simulink model "Observador"  (R2019a)
settings: Solver=VariableStepAuto  StartTime=0.0  StopTime=5  RelTol=1e-3
values from neighbouring files (symbols this model uses):
  A = [0 1 0;42.5 0 20;0 0 -4]    [Berard_Modelo_ControlEE.m]
  B = [0 0 1]'    [Berard_Modelo_ControlEE.m]
  C = k*C    [Berard_LoopShaping.m]    (also in Berard_Modelo_ControlEE.m = [1 0 0])
  k_g = k_a(1:3)    [Berard_Modelo_ControlEE.m]
  k_i = -k_a(end)    [Berard_Modelo_ControlEE.m]
  L = R*C*H*M    [Berard_LoopShaping.m]    (also in Berard_Modelo_ControlEE.m = acker(A',C',[-70 -70 -70])')
settings Model: Creator=agusd  LastModifiedBy=ARLUBER1
settings DataIOCC: ReturnWorkspaceOutputs=off
settings DebuggingCC: ArithmeticOperatorsInVariantConditions=warning
settings SFSimCC: SimUseLocalCustomCode=off
settings RTWCC: RTWUseLocalCustomCode=off
settings CodeAppCC: StateflowObjectComments=on

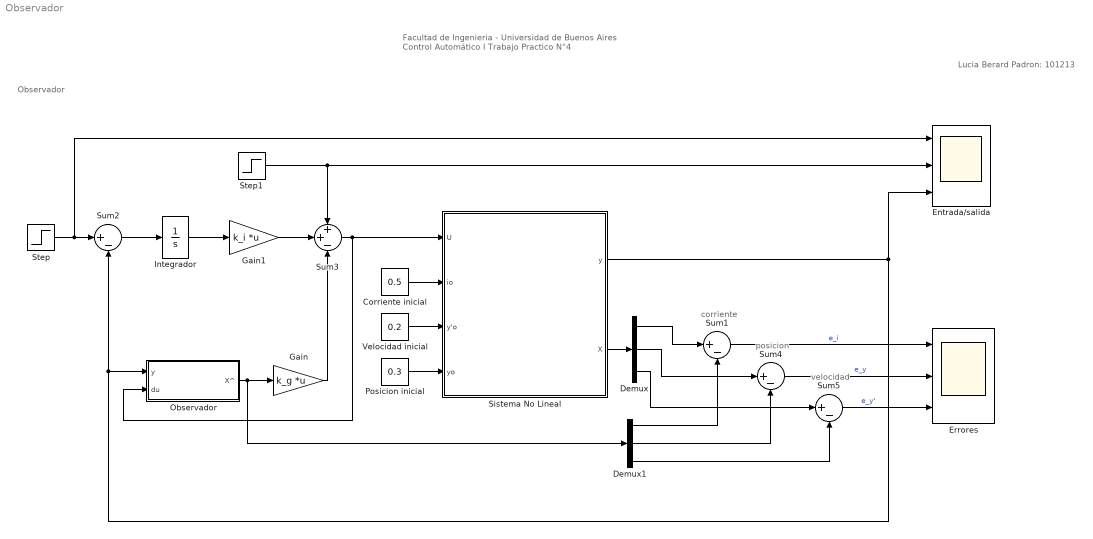
== system Observador ==
  note: velocidad
  note: posicion
  note: corriente
  note: Lucia Berard
      | Padron: 101213
  note: Observador
  note: Facultad de Ingenieria - Universidad de Buenos Aires
      | Control Automático I
      | Trabajo Practico N°4
  Corriente inicial : Constant  Value=0.5
  Demux : Demux  Outputs=3
  Demux1 : Demux  Outputs=3
  Entrada/salida : Scope  NumInputPorts=3
  Errores : Scope  NumInputPorts=3
  Gain : Gain  Gain=k_g  Multiplication=Matrix(K*u)
  Gain1 : Gain  Gain=k_i  Multiplication=Matrix(K*u)
  Integrador : Integrator
  Observador : Subsystem
  Posicion inicial : Constant  Value=0.3
  Sistema No Lineal : Subsystem
  Step : Step  After=0.5  SampleTime=0
  Step1 : Step  Time=3  After=0.55  SampleTime=0
  Sum{1..2,4..5} (4 alike) : Sum  Inputs=|+-
  Sum3 : Sum  Inputs=++-
  Velocidad inicial : Constant  Value=0.2
  wires:
  Corriente inicial/1 -> Sistema No Lineal/2(io)
  Velocidad inicial/1 -> Sistema No Lineal/3(y'o)
  Posicion inicial/1 -> Sistema No Lineal/4(yo)
  Step/1 -> Entrada/salida/1, Sum2/1
  Sum2/1 -> Integrador/1
  Integrador/1 -> Gain1/1
  Sum3/1 -> Observador/2(du), Sistema No Lineal/1(U)
  Sistema No Lineal/1("y ") -> Observador/1(y), Sum2/2, Entrada/salida/3
  Step1/1 -> Sum3/1, Entrada/salida/2
  Gain1/1 -> Sum3/2
  Observador/1(X^) -> Demux1/1, Gain/1
  Gain/1 -> Sum3/3
  Sum1/1 -> Errores/1  "e_i"
  Sum4/1 -> Errores/2  "e_y"
  Sum5/1 -> Errores/3  "e_y'"
  Sistema No Lineal/2(X) -> Demux/1
  Demux/1 -> Sum1/1
  Demux/2 -> Sum4/1
  Demux/3 -> Sum5/1
  Demux1/1 -> Sum1/2
  Demux1/2 -> Sum4/2
  Demux1/3 -> Sum5/2

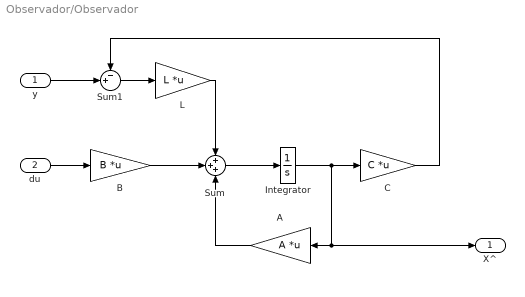
== system Observador/Observador ==
  y : Inport
  du : Inport  Port=2
  A : Gain  Gain=A  Multiplication=Matrix(K*u)
  B : Gain  Gain=B  Multiplication=Matrix(K*u)
  C : Gain  Gain=C  Multiplication=Matrix(K*u)
  Integrator : Integrator
  L : Gain  Gain=L  Multiplication=Matrix(K*u)
  Sum : Sum  Inputs=+++
  Sum1 : Sum  Inputs=-+|
  X^ : Outport
  wires:
  du/1 -> B/1
  Integrator/1 -> A/1, X^/1, C/1
  y/1 -> Sum1/2
  Sum1/1 -> L/1
  B/1 -> Sum/2
  A/1 -> Sum/3
  Sum/1 -> Integrator/1
  L/1 -> Sum/1
  C/1 -> Sum1/1

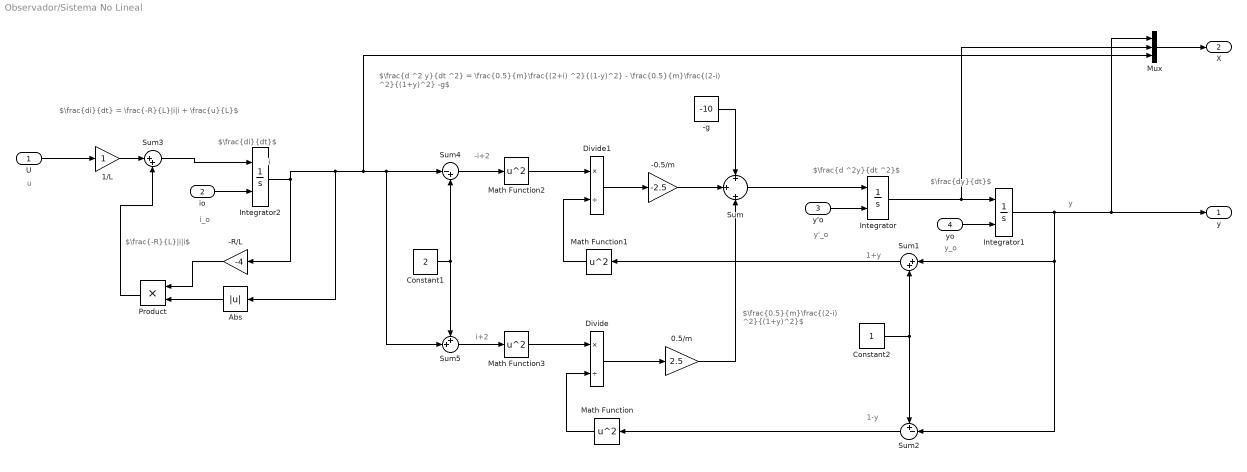
== system Observador/Sistema No Lineal ==
  note: y_o
  note: 1+y
  note: $\frac{di}{dt}$
  note: u
  note: i+2
  note: $\frac{d ^2 y}{dt ^2} = \frac{0.5}{m}\frac{(2+i) ^2}{(1-y)^2} - \frac{0.5}{m}\frac{(2-i) ^2}{(1+y)^2} -g$
  note: y
  note: 1-y
  note: i_o
  note: $\frac{dy}{dt}$
  note: y'_o
  note: $\frac{di}{dt} = \frac{-R}{L}|i|i + \frac{u}{L}$
  note: -i+2
  note: $\frac{-R}{L}|i|i$
  note: i
  note: $\frac{0.5}{m}\frac{(2-i) ^2}{(1+y)^2}$
  note: $\frac{d ^2y}{dt ^2}$
  U : Inport  OutDataTypeStr=double
  io : Inport  Port=2  OutDataTypeStr=double
  y'o : Inport  Port=3
  yo : Inport  Port=4
  -0.5/m : Gain  Gain=-2.5
  -R/L : Gain  Gain=-4
  -g : Constant  Value=-10
  0.5/m : Gain  Gain=2.5
  1/L : Gain
  Abs : Abs
  Constant1 : Constant  Value=2
  Constant2 : Constant
  Divide : Product  Inputs=*/
  Divide1 : Product  Inputs=*/
  Integrator : Integrator  InitialConditionSource=external
  Integrator1 : Integrator  InitialConditionSource=external  UpperSaturationLimit=1  LowerSaturationLimit=-1
  Integrator2 : Integrator  InitialConditionSource=external
  Math Function{,1..3} (4 alike) : Math  Operator=square  SaturateOnIntegerOverflow=on
  Mux : Mux  Inputs=3
  Product : Product
  Sum : Sum  Inputs=+|+|+
  Sum1 : Sum  Inputs=|++
  Sum2 : Sum  Inputs=+-|
  Sum3 : Sum  Inputs=|++
  Sum4 : Sum  Inputs=|-+
  Sum5 : Sum  Inputs=++|
  "y " : Outport
  X : Outport  Port=2
  wires:
  Divide1/1 -> -0.5/m/1
  -0.5/m/1 -> Sum/2
  Math Function2/1 -> Divide1/1
  Integrator/1 -> Mux/2, Integrator1/1
  Sum5/1 -> Math Function3/1
  Sum4/1 -> Math Function2/1
  -R/L/1 -> Product/1
  io/1 -> Integrator2/2
  Sum2/1 -> Math Function/1
  U/1 -> 1/L/1
  Sum/1 -> Integrator/1
  Math Function1/1 -> Divide1/2
  Sum3/1 -> Integrator2/1
  0.5/m/1 -> Sum/3
  Constant1/1 -> Sum4/2, Sum5/1
  Product/1 -> Sum3/2
  y'o/1 -> Integrator/2
  Abs/1 -> Product/2
  1/L/1 -> Sum3/1
  Integrator1/1 -> Mux/1, "y "/1, Sum1/1, Sum2/2
  Constant2/1 -> Sum2/1, Sum1/2
  Mux/1 -> X/1
  Divide/1 -> 0.5/m/1
  yo/1 -> Integrator1/2
  -g/1 -> Sum/1
  Integrator2/1 -> Mux/3, Sum5/2, Sum4/1, Abs/1, -R/L/1
  Sum1/1 -> Math Function1/1
  Math Function/1 -> Divide/2
  Math Function3/1 -> Divide/1
